simulink model "Hinf"  (R2025b)
settings: Solver=VariableStepAuto  StartTime=0.0  StopTime=1e3  RelTol=1e-3
libraries: cstblocks x2
settings Model: Creator=inggi  LastModifiedBy=inggi

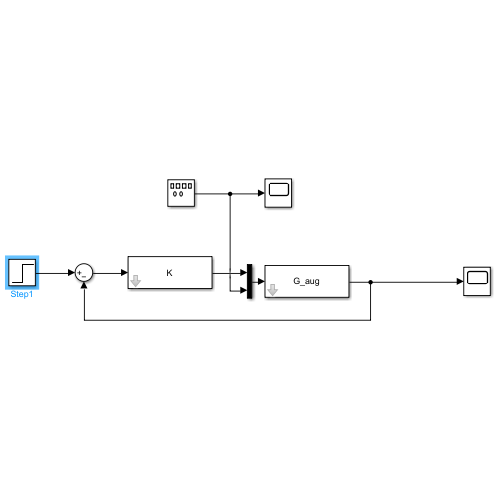
[thumbnail: Simulink's stored preview of the top-level diagram]
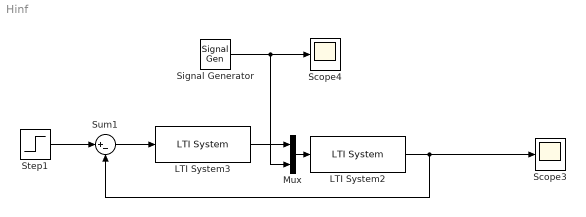
== system Hinf ==
  LTI System2 : cstblocks/LTI System  sys=G_aug  IC=[]  PadeOrder=0
  LTI System3 : cstblocks/LTI System  sys=K  IC=[]  PadeOrder=0
  Mux : Mux  Inputs=2
  Scope3 : Scope
      settings: ActiveDisplayYMinimum=-0.749833988412586  ActiveDisplayYMaximum=-0.12722698848597236
  Scope4 : Scope
      settings: ActiveDisplayYMinimum=-0.50833  ActiveDisplayYMaximum=3.36794  DataLoggingVariableName=ScopeData2
  Signal Generator : SignalGenerator  Frequency=10  Units=rad/sec
  Step1 : Step  Time=0  Before=zeros(1,5)  After=ones(1,5)  SampleTime=0
  Sum1 : Sum  Inputs=|+-
  wires:
  LTI System2/1 -> Scope3/1, Sum1/2
  LTI System3/1 -> Mux/1
  Sum1/1 -> LTI System3/1
  Step1/1 -> Sum1/1
  Signal Generator/1 -> Scope4/1, Mux/2
  Mux/1 -> LTI System2/1
